simulink model "rotor"  (R2024a)
settings: Solver=ode5  StartTime=0.0  StopTime=inf  FixedStep=SampleTime  RelTol=1e-3
values from neighbouring files (symbols this model uses):
  Arm = [ ... (first row only)    [launch.m]
  CDval = 0.008    [launch.m]
  g = 9.81    [launch.m]
  m = 1    [launch.m]
  m_to_mm = 1000    [launch.m]
  prop_inertia = (1/12) * 0.015 * 0.127^2    (= 2.016125e-05)    [launch.m]
  R = 0.127    [launch.m]
  SampleTime = 0.01    [launch.m]
  tilt_speed = [0; pi/4; 0]    [launch.m]
undefined symbols (not defined in the file or in its folder): ddx, ddy, ddz, dx, dy, dz, fractalcoef, lastVh, p, pitch, q, r, roll, X, Y, yaw, Z
libraries: simulink x4, sharedutil x3, aerolibatmos2 x1, sensorgpslib x1, robotcorelib x1, mspsensorlib x1, aerolibanimutils x1, shared6dof x1, simulink_extras x1, matrix_library x1, uavutilslib x1
(part 2 of 2)

== system rotor/Subsystem/Airframe/Motor Forces and Torques/If non tilted/Multirotor Subsystem/Rotor Subsystem/Non Tilted Ct estimator/Ct//C0 State Switcher/Descent ==
  In1 : Inport
  Action Port : ActionPort  ActionPortLabel=if(u1 >= -2 & u1 <= 0)
  Out1 : Outport
  wires:
  In1/1 -> Out1/1

== system rotor/Subsystem/Airframe/Motor Forces and Torques/If non tilted/Multirotor Subsystem/Rotor Subsystem/Non Tilted Ct estimator/Ct//C0 State Switcher/Past Curve Fit ==
  note: 1/2*ln(-(x+1.7439783573836165)) + 2.07884583669
  " Vz/Vh" : Inport
  Action Port : ActionPort  ActionPortLabel=elseif(u1 < -2)
  Add : Sum
  Constant : Constant  Value=2.07884583669
  Constant1 : Constant  Value=1.7439783573836165
  Gain : Gain  Gain=1/2
  Multiply : Gain  Gain=-1
  Sum : Sum  Inputs=|++
  ln : Math  Operator=log
  " " : Outport
  wires:
  Add/1 -> " "/1
  Constant/1 -> Add/2
  Multiply/1 -> ln/1
  ln/1 -> Gain/1
  " Vz/Vh"/1 -> Sum/1
  Sum/1 -> Multiply/1
  Constant1/1 -> Sum/2
  Gain/1 -> Add/1

== system rotor/Subsystem/Airframe/Motor Forces and Torques/If transitioning/Multirotor Subsystem/Rotor Subsystem/Tilted Ct Estimator/Ct//C0 State Switcher/If Action Subsystem ==
  In1 : Inport
  Action Port : ActionPort  ActionPortLabel=if(u1 >= -2.828427125 & u1 <= 0)
  Out1 : Outport
  wires:
  In1/1 -> Out1/1

== system rotor/Subsystem/Airframe/Motor Forces and Torques/If transitioning/Multirotor Subsystem/Rotor Subsystem/Tilted Ct Estimator/Ct//C0 State Switcher/If Action Subsystem1 ==
  " Vz/Vh" : Inport
  Action Port : ActionPort  ActionPortLabel=elseif(u1 < -2.828427125)
  Add : Sum
  Constant : Constant  Value=1.007639046
  Multiply : Gain  Gain=-1
  ln : Math  Operator=log
  " " : Outport
  wires:
  Add/1 -> " "/1
  Constant/1 -> Add/2
  Multiply/1 -> ln/1
  " Vz/Vh"/1 -> Multiply/1
  ln/1 -> Add/1

== system rotor/Subsystem/Airframe/Motor Forces and Torques/If transitioning/Multirotor Subsystem/Rotor Subsystem/Tilted Ct Estimator/Ct//C0 State Switcher/If Action Subsystem2 ==
  "  " : Inport
  Action Port : ActionPort  ActionPortLabel=else
  Out1 : Outport
  wires:
  "  "/1 -> Out1/1

== matlab function rotor/Subsystem/Airframe/Motor Forces and Torques/If transitioning/Multirotor Subsystem/Rotor Subsystem/Induced Vel Convergence Checker ==
  data: rpmToCalc output; newVh output; Converged output; Vh input; convergence_threshold parameter; lastVh input
function [rpmToCalc, newVh, Converged] = CalculateInducedVelocity(Vh, convergence_threshold, lastVh)

    % Initialize variables
    persistent rpm_index rpm_values Vh_values exportedCoefficients;

    if isempty(rpm_index)
        rpm_index = 1;
        rpm_values = 1:1000:10001;
        Vh_values = zeros(size(rpm_values));
        exportedCoefficients = false;
    end

    if rpm_index > 11
        rpmToCalc = 1;
        newVh = 0.1;
        Converged = 1;
        return;
    end

    % Calculate the difference between the current and last induced velocity
    difference = abs(Vh - lastVh);
    rpmToCalc = rpm_values(rpm_index);

    if difference < convergence_threshold
        % Convergence achieved
        Converged = 1;
        newVh = Vh; % Update to the current induced velocity
        Vh_values(rpm_index) = Vh;
        
        if rpm_index >= length(rpm_values) && exportedCoefficients == false
            coefficients = fitVhToRPM(rpm_values, Vh_values);
            assignin('base', 'coefficients', coefficients);
            assignin('base', 'rpm_values', rpm_values);
            assignin('base', 'Vh_values', Vh_values);
            exportedCoefficients = true;
            return;
        else
            if rpm_index ~= 11
                rpmToCalc = rpm_values(rpm_index+1);
            end
        end

        % Move to the next RPM value
        if rpm_index < 11
            rpm_index = rpm_index + 1;
        end
    else
        % Convergence not achieved
        Converged = 0;
        newVh = Vh; % Update to the new induced velocity
    end
end

function coefficients = fitVhToRPM(rpm_values, Vh_values)
    % Fit a polynomial (or any other function) to the RPM and Vh values
    p = polyfit(rpm_values, Vh_values, 2);
    coefficients = p;
end

== matlab function rotor/Subsystem/Airframe/Motor Forces and Torques/If non tilted/Multirotor Subsystem/Rotor Subsystem/Induced Vel Convergence Checker ==
  data: rpmToCalc output; newVh output; Converged output; Vh input; convergence_threshold parameter; lastVh input
function [rpmToCalc, newVh, Converged] = CalculateInducedVelocity(Vh, convergence_threshold, lastVh)

    % Initialize variables
    persistent rpm_index rpm_values Vh_values exportedCoefficients;

    if isempty(rpm_index)
        rpm_index = 1;
        rpm_values = 1:1000:10001;
        Vh_values = zeros(size(rpm_values));
        exportedCoefficients = false;
    end

    if rpm_index > 11
        rpmToCalc = 1;
        newVh = 0.1;
        Converged = 1;
        return;
    end

    % Calculate the difference between the current and last induced velocity
    difference = abs(Vh - lastVh);
    rpmToCalc = rpm_values(rpm_index);

    if difference < convergence_threshold
        % Convergence achieved
        Converged = 1;
        newVh = Vh; % Update to the current induced velocity
        Vh_values(rpm_index) = Vh;
        
        if rpm_index >= length(rpm_values) && exportedCoefficients == false
            coefficients = fitVhToRPM(rpm_values, Vh_values);
            assignin('base', 'coefficients', coefficients);
            assignin('base', 'rpm_values', rpm_values);
            assignin('base', 'Vh_values', Vh_values);
            exportedCoefficients = true;
            return;
        else
            if rpm_index ~= 11
                rpmToCalc = rpm_values(rpm_index+1);
            end
        end

        % Move to the next RPM value
        if rpm_index < 11
            rpm_index = rpm_index + 1;
        end
    else
        % Convergence not achieved
        Converged = 0;
        newVh = Vh; % Update to the new induced velocity
    end
end

function coefficients = fitVhToRPM(rpm_values, Vh_values)
    % Fit a polynomial (or any other function) to the RPM and Vh values
    p = polyfit(rpm_values, Vh_values, 2);
    coefficients = p;
end

== matlab function rotor/Subsystem/Airframe/Motor Forces and Torques/If Tilted/Multirotor Subsystem/Rotor Subsystem/Induced Vel Convergence Checker ==
  data: rpmToCalc output; newVh output; Converged output; Vh input; convergence_threshold parameter; lastVh input
function [rpmToCalc, newVh, Converged] = CalculateInducedVelocity(Vh, convergence_threshold, lastVh)

    % Initialize variables
    persistent rpm_index rpm_values Vh_values exportedCoefficients;

    if isempty(rpm_index)
        rpm_index = 1;
        rpm_values = 1:1000:10001;
        Vh_values = zeros(size(rpm_values));
        exportedCoefficients = false;
    end

    if rpm_index > 11
        rpmToCalc = 1;
        newVh = 0.1;
        Converged = 1;
        return;
    end

    % Calculate the difference between the current and last induced velocity
    difference = abs(Vh - lastVh);
    rpmToCalc = rpm_values(rpm_index);

    if difference < convergence_threshold
        % Convergence achieved
        Converged = 1;
        newVh = Vh; % Update to the current induced velocity
        Vh_values(rpm_index) = Vh;
        
        if rpm_index >= length(rpm_values) && exportedCoefficients == false
            coefficients = fitVhToRPM(rpm_values, Vh_values);
            assignin('base', 'coefficients', coefficients);
            assignin('base', 'rpm_values', rpm_values);
            assignin('base', 'Vh_values', Vh_values);
            exportedCoefficients = true;
            return;
        else
            if rpm_index ~= 11
                rpmToCalc = rpm_values(rpm_index+1);
            end
        end

        % Move to the next RPM value
        if rpm_index < 11
            rpm_index = rpm_index + 1;
        end
    else
        % Convergence not achieved
        Converged = 0;
        newVh = Vh; % Update to the new induced velocity
    end
end

function coefficients = fitVhToRPM(rpm_values, Vh_values)
    % Fit a polynomial (or any other function) to the RPM and Vh values
    p = polyfit(rpm_values, Vh_values, 2);
    coefficients = p;
end
